simulink model "ifelseifBlock"  (R2023b)
settings: Solver=VariableStepAuto  StartTime=0.0  StopTime=10.0  RelTol=1e-3

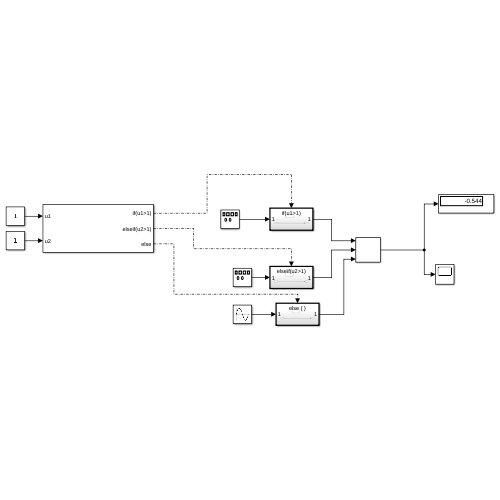
[thumbnail: Simulink's stored preview of the top-level diagram]
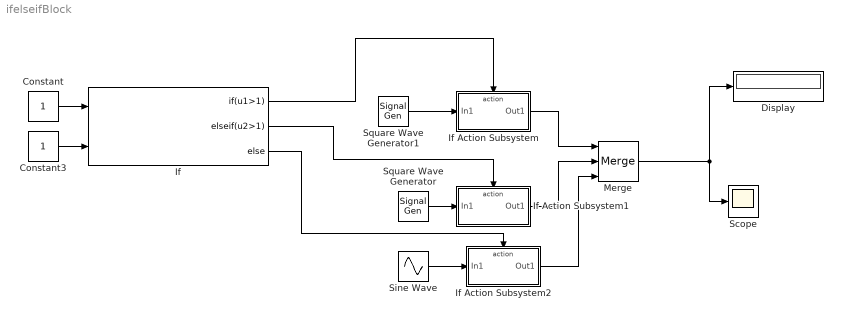
== system ifelseifBlock ==
  Constant : Constant
  Constant3 : Constant
  Display : Display
  If : If  NumInputs=2  IfExpression=u1>1  ElseIfExpressions=u2>1
  If Action Subsystem : Subsystem  TreatAsAtomicUnit=on
  If Action Subsystem1 : Subsystem  TreatAsAtomicUnit=on
  If Action Subsystem2 : Subsystem  TreatAsAtomicUnit=on
  Merge : Merge  Inputs=3
  Scope : Scope
  Sine Wave : Sin  SampleTime=0
  Square Wave Generator : SignalGenerator  WaveForm=square  Frequency=100  Units=rad/sec
  Square Wave Generator1 : SignalGenerator  WaveForm=square  Frequency=10  Units=rad/sec
  wires:
  Constant/1 -> If/1
  If/1 -> If Action Subsystem/Action
  If Action Subsystem/1(Out1) -> Merge/1
  If Action Subsystem1/1(Out1) -> Merge/2
  Merge/1 -> Scope/1, Display/1
  Constant3/1 -> If/2
  If/2 -> If Action Subsystem1/Action
  If/3 -> If Action Subsystem2/Action
  Square Wave Generator/1 -> If Action Subsystem1/1(In1)
  Sine Wave/1 -> If Action Subsystem2/1(In1)
  Square Wave Generator1/1 -> If Action Subsystem/1(In1)
  If Action Subsystem2/1(Out1) -> Merge/3

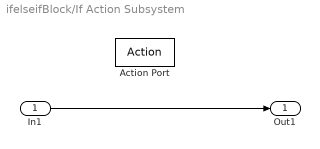
== system ifelseifBlock/If Action Subsystem ==
  In1 : Inport
  Action Port : ActionPort  ActionPortLabel=if(u1>1)
  Out1 : Outport
  wires:
  In1/1 -> Out1/1

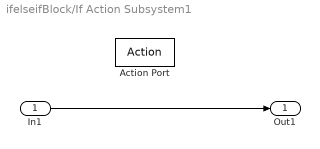
== system ifelseifBlock/If Action Subsystem1 ==
  In1 : Inport
  Action Port : ActionPort  ActionPortLabel=elseif(u2>1)
  Out1 : Outport
  wires:
  In1/1 -> Out1/1

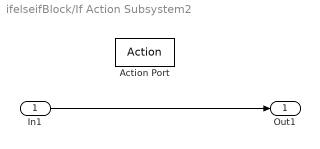
== system ifelseifBlock/If Action Subsystem2 ==
  In1 : Inport
  Action Port : ActionPort  ActionPortLabel=else
  Out1 : Outport
  wires:
  In1/1 -> Out1/1
